simulink subsystem "sub1"  (R2020a)
settings: Solver=VariableStepAuto  StartTime=0.0  StopTime=10.0  RelTol=1e-3
libraries: simulink x4
settings Model: Creator=ecs  LastModifiedBy=ecs

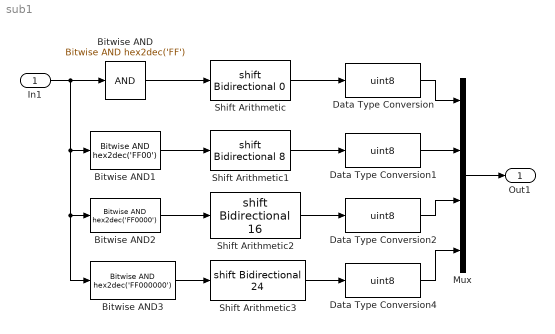
== system sub1 ==
  In1 : Inport  OutDataTypeStr=uint32
  Bitwise AND : simulink/Logic and Bit Operations/Bitwise Operator  logicop=AND  UseBitMask=on  BitMask=hex2dec('FF')  BitMaskRealWorld=Stored Integer
  Bitwise AND1 : simulink/Logic and Bit Operations/Bitwise Operator  logicop=AND  UseBitMask=on  BitMask=hex2dec('FF00')  BitMaskRealWorld=Stored Integer
  Bitwise AND2 : simulink/Logic and Bit Operations/Bitwise Operator  logicop=AND  UseBitMask=on  BitMask=hex2dec('FF0000')  BitMaskRealWorld=Stored Integer
  Bitwise AND3 : simulink/Logic and Bit Operations/Bitwise Operator  logicop=AND  UseBitMask=on  BitMask=hex2dec('FF000000')  BitMaskRealWorld=Stored Integer
  Data Type Conversion{,1..2,4} (4 alike) : DataTypeConversion  OutDataTypeStr=uint8
  Mux : Mux
  Shift Arithmetic : ArithShift
  Shift Arithmetic1 : ArithShift  BitShiftNumber=8
  Shift Arithmetic2 : ArithShift  BitShiftNumber=16
  Shift Arithmetic3 : ArithShift  BitShiftNumber=24
  Out1 : Outport
  wires:
  Bitwise AND3/1 -> Shift Arithmetic3/1
  In1/1 -> Bitwise AND2/1, Bitwise AND3/1, Bitwise AND1/1, Bitwise AND/1
  Bitwise AND2/1 -> Shift Arithmetic2/1
  Bitwise AND1/1 -> Shift Arithmetic1/1
  Data Type Conversion1/1 -> Mux/2
  Mux/1 -> Out1/1
  Shift Arithmetic2/1 -> Data Type Conversion2/1
  Shift Arithmetic3/1 -> Data Type Conversion4/1
  Shift Arithmetic1/1 -> Data Type Conversion1/1
  Data Type Conversion4/1 -> Mux/4
  Bitwise AND/1 -> Shift Arithmetic/1
  Data Type Conversion2/1 -> Mux/3
  Data Type Conversion/1 -> Mux/1
  Shift Arithmetic/1 -> Data Type Conversion/1
